simulink model "VCU_Modes_UnitTest"  (R2025b)
settings: Solver=FixedStepDiscrete  StartTime=0.0  StopTime=11  RelTol=1e-3
settings Model: Creator=2503-00091  LastModifiedBy=2503-00091
settings OptimizationCC: DefaultParameterBehavior=Inlined  EnhancedBackFolding=on  PassReuseOutputArgsAs=Individual arguments  ZeroExternalMemoryAtStartup=off  ZeroInternalMemoryAtStartup=off  OptimizeBlockOrder=speed  DifferentSizesBufferReuse=on  OptimizationCustomize=off  LabelGuidedReuse=on  EfficientTunableParamExpr=on
settings DebuggingCC: AlgebraicLoopMsg=error  ArtificialAlgebraicLoopMsg=error  ParameterTunabilityLossMsg=error  UnitsInconsistencyMsg=none
settings HardwareCC: TargetBitPerPointer=64.0  TargetBitPerSizeT=64.0  TargetBitPerPtrDiffT=64.0  TargetLargestAtomicFloat=Float  TargetIntDivRoundTo=Zero  TargetEndianess=LittleEndian  TargetWordSize=64.0  TargetHWDeviceType=Intel->x86-64 (Windows64)  ProdEqTarget=off
settings SFSimCC: MATLABDynamicMemAlloc=off
settings RTWCC: SystemTargetFile=ert.tlc  TemplateMakefile=ert_default_tmf  Description=Embedded Coder
settings CodeAppCC: ForceParamTrailComments=on  IgnoreCustomStorageClasses=off  OperatorAnnotations=on  SimulinkDataObjDesc=on  SFDataObjDesc=on  InsertBlockDesc=on
settings ERTTargetCC: ERTCustomFileTemplate=example_file_process.tlc  TargetLangStandard=C99 (ISO)  GenerateSampleERTMain=on

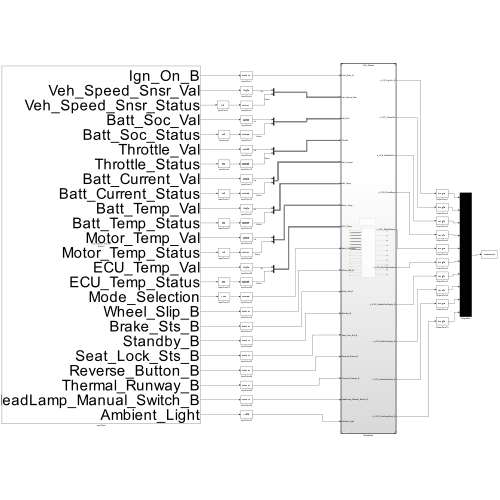
[thumbnail: Simulink's stored preview of the top-level diagram]
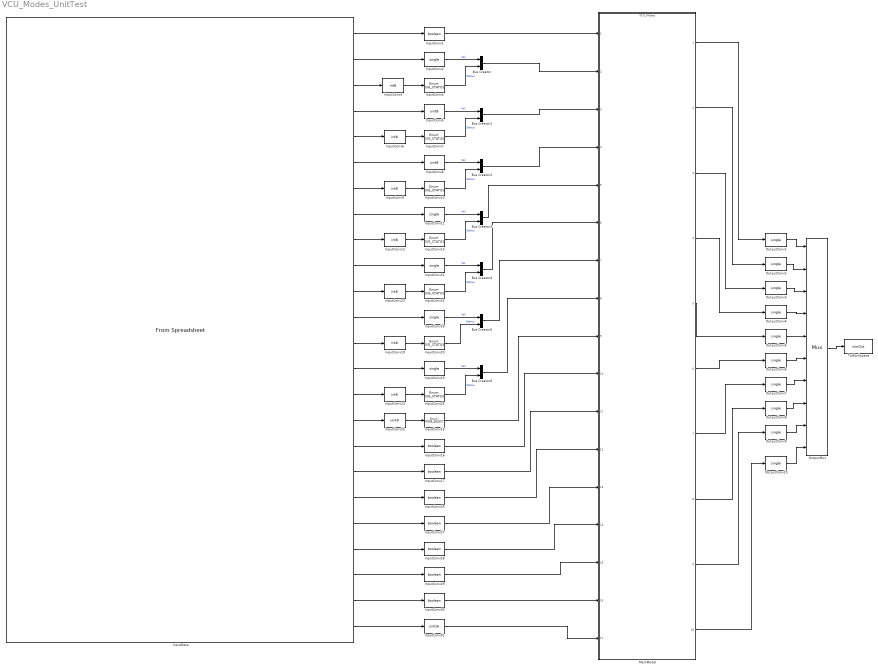
== system VCU_Modes_UnitTest ==
  Bus Creator{,1..6} (7 alike) : BusCreator  Inputs=2
  InputConv{1,16..17,26..30} (8 alike) : DataTypeConversion  OutDataTypeStr=boolean  SaturateOnIntegerOverflow=off  RndMeth=Floor
  InputConv{4,7,10,13..14,20,25} (7 alike) : DataTypeConversion  OutDataTypeStr=Enum: SIG_STATUS  SaturateOnIntegerOverflow=off  RndMeth=Floor
  InputConv{2,11,18,21,23} (5 alike) : DataTypeConversion  OutDataTypeStr=single  SaturateOnIntegerOverflow=off  RndMeth=Floor
  InputConv{3,6,9,12,19,22,24} (7 alike) : DataTypeConversion  OutDataTypeStr=int8  SaturateOnIntegerOverflow=off  RndMeth=Floor
  InputConv15 : DataTypeConversion  OutDataTypeStr=Enum: MODE_SELECT  SaturateOnIntegerOverflow=off  RndMeth=Floor
  InputConv31 : DataTypeConversion  OutDataTypeStr=uint16  SaturateOnIntegerOverflow=off  RndMeth=Floor
  InputConv32 : DataTypeConversion  OutDataTypeStr=uint8  SaturateOnIntegerOverflow=off  RndMeth=Floor
  InputConv5 : DataTypeConversion  OutDataTypeStr=uint8  SaturateOnIntegerOverflow=off  RndMeth=Floor
  InputConv8 : DataTypeConversion  OutDataTypeStr=uint8  SaturateOnIntegerOverflow=off  RndMeth=Floor
  InputData : FromSpreadsheet  FileName=VCU_Modes_Test.xlsx
  MainModel : ModelReference  ModelNameDialog=VCU_Modes  SimulationMode=Normal  ModelReferenceVersion=1.105
  OutputConv{1..10} (10 alike) : DataTypeConversion  OutDataTypeStr=single  SaturateOnIntegerOverflow=off  RndMeth=Floor
  OutputMux : Mux  Inputs=10
  ToWorkspace : ToWorkspace  VariableName=simOut  SaveFormat=Structure With Time  SampleTime=-1
  wires:
  InputData/1 -> InputConv1/1
  MainModel/1 -> OutputConv1/1
  OutputConv1/1 -> OutputMux/1
  MainModel/2 -> OutputConv2/1
  OutputConv2/1 -> OutputMux/2
  MainModel/3 -> OutputConv3/1
  OutputConv3/1 -> OutputMux/3
  MainModel/4 -> OutputConv4/1
  OutputConv4/1 -> OutputMux/4
  MainModel/5 -> OutputConv5/1
  OutputConv5/1 -> OutputMux/5
  MainModel/6 -> OutputConv6/1
  OutputConv6/1 -> OutputMux/6
  MainModel/7 -> OutputConv7/1
  OutputConv7/1 -> OutputMux/7
  MainModel/8 -> OutputConv8/1
  OutputConv8/1 -> OutputMux/8
  MainModel/9 -> OutputConv9/1
  OutputConv9/1 -> OutputMux/9
  OutputMux/1 -> ToWorkspace/1
  InputConv1/1 -> MainModel/1
  InputData/2 -> InputConv2/1
  InputData/3 -> InputConv3/1
  InputConv3/1 -> InputConv4/1
  InputConv2/1 -> Bus Creator/1  "Val"
  InputConv4/1 -> Bus Creator/2  "Status"
  Bus Creator/1 -> MainModel/2
  InputData/5 -> InputConv6/1
  InputData/4 -> InputConv5/1
  InputConv7/1 -> Bus Creator1/2  "Status"
  InputConv6/1 -> InputConv7/1
  InputConv5/1 -> Bus Creator1/1  "Val"
  Bus Creator1/1 -> MainModel/3
  InputData/9 -> InputConv12/1
  InputData/8 -> InputConv11/1
  Bus Creator2/1 -> MainModel/4
  InputConv11/1 -> Bus Creator3/1  "Val"
  InputConv12/1 -> InputConv13/1
  InputData/7 -> InputConv9/1
  InputConv13/1 -> Bus Creator3/2  "Status"
  InputData/6 -> InputConv8/1
  InputConv10/1 -> Bus Creator2/2  "Status"
  Bus Creator3/1 -> MainModel/5
  InputConv8/1 -> Bus Creator2/1  "Val"
  InputConv9/1 -> InputConv10/1
  Bus Creator4/1 -> MainModel/6
  Bus Creator5/1 -> MainModel/7
  InputConv22/1 -> InputConv14/1
  InputConv21/1 -> Bus Creator4/1  "Val"
  InputConv14/1 -> Bus Creator4/2  "Status"
  InputConv18/1 -> Bus Creator5/1  "Val"
  InputConv20/1 -> Bus Creator5/2  "Status"
  InputConv19/1 -> InputConv20/1
  InputData/12 -> InputConv18/1
  InputData/10 -> InputConv21/1
  InputData/13 -> InputConv19/1
  InputData/11 -> InputConv22/1
  Bus Creator6/1 -> MainModel/8
  InputData/14 -> InputConv23/1
  InputConv25/1 -> Bus Creator6/2  "Status"
  InputConv24/1 -> InputConv25/1
  InputData/15 -> InputConv24/1
  InputConv23/1 -> Bus Creator6/1  "Val"
  InputConv15/1 -> MainModel/9
  InputData/16 -> InputConv32/1
  InputData/17 -> InputConv16/1
  InputData/18 -> InputConv17/1
  InputData/19 -> InputConv26/1
  InputConv26/1 -> MainModel/12
  InputConv17/1 -> MainModel/11
  InputConv16/1 -> MainModel/10
  InputData/20 -> InputConv27/1
  InputData/21 -> InputConv28/1
  InputData/22 -> InputConv29/1
  InputConv29/1 -> MainModel/15
  InputConv28/1 -> MainModel/14
  InputConv27/1 -> MainModel/13
  InputConv30/1 -> MainModel/16
  InputData/23 -> InputConv30/1
  InputData/24 -> InputConv31/1
  InputConv31/1 -> MainModel/17
  InputConv32/1 -> InputConv15/1
  OutputConv10/1 -> OutputMux/10
  MainModel/10 -> OutputConv10/1
